simulink model "simulink_filter"  (Simulink 9.1)
settings: Solver=FixedStepDiscrete  StartTime=0.0  StopTime=inf  RelTol=1e-3
values from neighbouring files (symbols this model uses):
  z = tf('z',Ts)    [adaptiveFilter.m]    (also in adaptivefilterNedret.m)
undefined symbols (not defined in the file or in its folder): k, p
settings Model: Creator=Heisenberg  LastModifiedBy=USER
settings SolverCC: AutoInsertRateTranBlk=on
settings DataIOCC: LimitDataPoints=on  SaveFormat=Dataset  SaveOutput=off  SignalLogging=off  DSMLogging=off  SaveTime=off
settings DebuggingCC: AlgebraicLoopMsg=error  UnderspecifiedInitializationDetection=Simplified  MergeDetectMultiDrivingBlocksExec=error  SingleTaskRateTransMsg=error  AllowSymbolicDim=off
settings HardwareCC: ProdBitPerPointer=64  ProdBitPerSizeT=64  ProdBitPerPtrDiffT=64  ProdLargestAtomicFloat=Float  ProdIntDivRoundTo=Zero  ProdEndianess=LittleEndian  ProdWordSize=64  ProdHWDeviceType=Intel->x86-64 (Windows64)
settings ModelReferenceCC: PropagateSignalLabelsOutOfModel=on
settings GRTTargetCC: GeneratePreprocessorConditionals=Disable all  CombineOutputUpdateFcns=on  GRTInterface=off
settings ConfigComp: CovMetricSettings=dwe  CovHtmlReporting=off  CovSaveCumulativeToWorkspaceVar=off  CovSaveSingleToWorkspaceVar=off  CovExternalEMLEnable=on

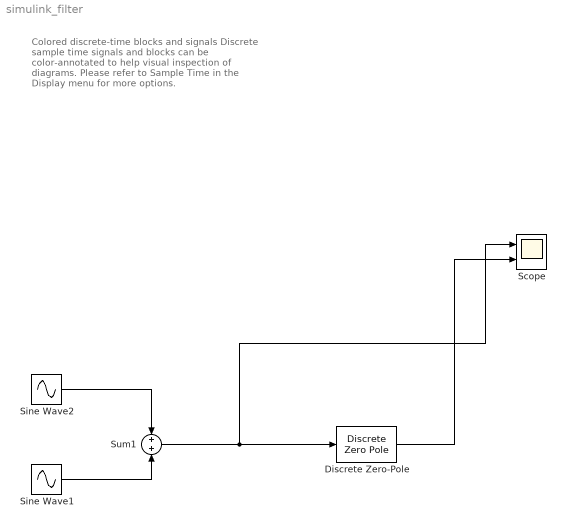
== system simulink_filter ==
  note: Colored discrete-time blocks and signals
      | Discrete sample time signals and blocks can be color-annotated to help visual inspection of diagrams. Please refer to Sample Time in the Display menu for more options.
  Discrete Zero-Pole : DiscreteZeroPole  Zeros=z  Poles=p  Gain=k  SampleTime=-1
  Scope : Scope  NumInputPorts=2
  Sine Wave1 : Sin  Frequency=2*pi*300  Samples=1  SampleTime=1/1000
  Sine Wave2 : Sin  Amplitude=5  Frequency=2*pi*50  Samples=1  SampleTime=1/1000
  Sum1 : Sum
  wires:
  Sine Wave1/1 -> Sum1/2
  Sum1/1 -> Discrete Zero-Pole/1, Scope/1
  Sine Wave2/1 -> Sum1/1
  Discrete Zero-Pole/1 -> Scope/2
